simulink model "A320"  (R2023b)
settings: Solver=ode4  StartTime=0.0  StopTime=150  FixedStep=0.001  RelTol=1e-3
values from neighbouring files (symbols this model uses):
  a0 = 340.294    [basedata.m]    (also in basedata.mat; control_design.mat; landing_init.m; landing_plan.mat)
  alpha_CL_table = [ -3.150;  0.000;  0.139;  0.200;  0.260;  0.290;  0.320;  0.500;  3.150 ]    [basedata.m]
  alpha_Cm_table = [ -3.150; -0.800; -0.400; -0.200; -0.100;  0.000;  0.200;  0.230;  0.260;  0.290;  0.310;  0.400;  0.800;  3.150 ]    [basedata.m]
  alpha_Kde_table = [ -3.141593; -0.698132; -0.349066; -0.174533; -0.087266;  0.000000;  0.087266;  0.174533;  0.349066;  0.698132;  3.141593 ]    [basedata.m]
  b_ref = 35.799979    [basedata.m]    (also in basedata.mat = 2; control_design.mat = 2; landing_init.m = 2; landing_plan.mat = 2)
  c_gear = [6.734e4, 1.179e5, 1.179e5]    [basedata.m]    (also in basedata.mat = [8000 14000 14000]; control_design.mat = [8000 14000 14000]; landing_init.m = [0.8e4, 1.4e4, 1.4e4]; landing_plan.mat = [8000 14000 14000])
  c_lat = [9.917e5, 1.852e6, 1.852e6]    [basedata.m]    (also in basedata.mat = [14000 22000 22000]; control_design.mat = [14000 22000 22000]; landing_init.m = [1.4e4, 2.2e4, 2.2e4]; landing_plan.mat = [14000 22000 22000])
  c_ref = S_ref / b_ref    (= 3.41891172618)    [basedata.m]    (also in basedata.mat = 0.9; control_design.mat = 0.9; landing_init.m = 0.9; landing_plan.mat = 0.9)
  c_roll = [0.020, 0.018, 0.018]    [basedata.m]    (also in basedata.mat = [0.02 0.018 0.018]; control_design.mat = [0.02 0.018 0.018]; landing_init.m; landing_plan.mat = [0.02 0.018 0.018])
  CD0 = 0.01865    [basedata.m]    (also in basedata.mat = 0.045; canshujisuan.m = 0.045; control_design.mat = 0.045; landing_init.m = 0.045)
  CL_D0 = CL_D0_clean    (= 0.175)    [basedata.m]
  CL_table = [  0.000;  0.138;  1.320;  1.480;  1.760;  1.750;  1.600;  1.500;  0.000 ]    [basedata.m]
  Clb = 0.554    [basedata.m]    (also in basedata.mat = -0.08; control_design.mat = -0.08; landing_init.m = -0.08; landing_plan.mat = -0.08)
  Clda = -0.291    [basedata.m]    (also in basedata.mat = -0.2; control_design.mat = -0.2; landing_init.m = -0.2; landing_plan.mat = -0.2)
  CLde = -1.652    [basedata.m]    (also in basedata.mat = 0.28; control_design.mat = 0.28; landing_init.m = 0.28; landing_plan.mat = 0.28)
  Cldr = 0.476    [basedata.m]
  Clp = -2.078    [basedata.m]    (also in basedata.mat = -0.7; control_design.mat = -0.7; landing_init.m = -0.7; landing_plan.mat = -0.7)
  CLq = -57.116    [basedata.m]    (also in basedata.mat = 4.5; canshujisuan.m = 3; control_design.mat = 4.5; landing_init.m = 4.5)
  Clr = -2.621    [basedata.m]    (also in basedata.mat = 0.08; control_design.mat = 0.08; landing_init.m = 0.08; landing_plan.mat = 0.08)
  Cm_table = [  0.000; -2.402; -1.861; -0.842; -0.442;  0.000;  1.173;  1.337;  1.489;  1.723;  1.919;  2.276;  2.992;  0.000 ]    [basedata.m]
  Cmde = -11.78    [basedata.m]    (also in basedata.mat = -0.9; control_design.mat = -0.9; landing_init.m = -0.9; landing_plan.mat = -0.9)
  Cmq = -1245.917    [basedata.m]    (also in basedata.mat = -18; control_design.mat = -18; landing_init.m = -18; landing_plan.mat = -18)
  Cnb = 1.296    [basedata.m]    (also in basedata.mat = 0.25; control_design.mat = 0.25; landing_init.m = 0.25; landing_plan.mat = 0.25)
  Cnda = -0.007    [basedata.m]
  Cndr = 1.321    [basedata.m]    (also in basedata.mat = -0.15; control_design.mat = -0.15; landing_init.m = -0.15; landing_plan.mat = -0.15)
  Cnp = 0.742    [basedata.m]    (also in basedata.mat = -0.04; control_design.mat = -0.04; landing_init.m = -0.04; landing_plan.mat = -0.04)
  Cnr = -67.303    [basedata.m]    (also in basedata.mat = -0.45; control_design.mat = -0.45; landing_init.m = -0.45; landing_plan.mat = -0.45)
  CSb = -3.252    [basedata.m]    (also in basedata.mat = -0.7; control_design.mat = -0.7; landing_init.m = -0.7; landing_plan.mat = -0.7)
  CSdr = -2.793    [basedata.m]    (also in basedata.mat = 0.18; control_design.mat = 0.18; landing_init.m = 0.18; landing_plan.mat = 0.18)
  CSr = 17.395    [basedata.m]    (also in basedata.mat = 0.12; control_design.mat = 0.12; landing_init.m = 0.12; landing_plan.mat = 0.12)
  CYp = 1.833    [basedata.m]
  D = 0.5 * rho0 * V^2 * S_ref * CD_current    [canshujisuan.m]
  D0 = 1400    [basedata.m]    (also in basedata.mat; control_design.mat = 800; landing.m; landing_init.m)
  da_max = 0.436332    [basedata.m]    (also in basedata.mat = 25; control_design.mat = 25; landing_init.m = 25; landing_plan.mat = 25)
  da_min = -da_max    (= -0.436332)    [basedata.m]    (also in basedata.mat = -25; control_design.mat = -25; landing_init.m = -25; landing_plan.mat = -25)
  de_max = 0.436332    [basedata.m]    (also in basedata.mat = 25; control_design.mat = 25; landing_init.m = 25; landing_plan.mat = 25)
  de_min = -0.296706    [basedata.m]    (also in basedata.mat = -25; control_design.mat = -25; landing_init.m = -25; landing_plan.mat = -25)
  Delta_CD_flap_tot = 0.1316    [basedata.m]
  Delta_CD_gear = 0.0372    [basedata.m]
  Delta_CD_sp = 0.05775    [basedata.m]
  Delta_CL_flap_tot = 1.867    [basedata.m]
  Delta_CL_sp = -0.466875    [basedata.m]
  Delta_Cm_flap_tot = -0.084    [basedata.m]
  Delta_Cm_gear = 0.0022    [basedata.m]
  Delta_Cm_sp = 0.023    [basedata.m]
  delta_flap_TE_max = 0.698132    [basedata.m]
  delta_flap_TE_tab = [ 0.000000;  0.087266;  0.174533;  0.261799;  0.349066;  0.698132 ]    [basedata.m]
  delta_slat_LE_max = 0.471239    [basedata.m]
  delta_slat_LE_tab = [ 0.000000;  0.314159;  0.314334;  0.383972;  0.384147;  0.471239 ]    [basedata.m]
  DH = pi / 180    (= 0.0174532925199)    [basedata.m]    (also in basedata.mat; control_design.mat; landing_init.m; landing_plan.mat)
  dr_max = 0.436332    [basedata.m]    (also in basedata.mat = 25; control_design.mat = 25; landing_init.m = 25; landing_plan.mat = 25)
  dr_min = -dr_max    (= -0.436332)    [basedata.m]    (also in basedata.mat = -25; control_design.mat = -25; landing_init.m = -25; landing_plan.mat = -25)
  g = 9.80665    [basedata.m]    (also in basedata.mat; canshujisuan.m; control_design.mat; landing_init.m)
  gD_flap_TE_tab = [ 0.000;     0.300;     0.630;     0.850;     0.970;     0.939 ]    [basedata.m]
  gD_slat_LE_tab = [ 1.000;     0.330;     0.630;     0.850;     0.970;     0.939 ]    [basedata.m]
  gL_flap_TE_tab = [ 0.000;     0.010;     1.300;     1.300;     1.170;     1.000 ]    [basedata.m]
  gL_slat_LE_tab = [ 1.000;     1.000;     1.000;     1.000;     1.000;     1.000 ]    [basedata.m]
  ground_z = 0.0    (= 0)    [basedata.m]    (also in basedata.mat; control_design.mat; landing_init.m; landing_plan.mat)
  H_B = 132.622761894    [basedata.mat]    (also in landing_trajectory.m = H_R - R * cos(a1); landingplan.mat)
  H_C = 72.1000994005    [basedata.mat]    (also in landing_trajectory.m = H_R - R * cos(a2); landingplan.mat)
  H_climb_complete = 1000    [control_design.mat]    (also in landing.m; landing_init.m; landing_plan.mat; landingplan.mat)
  H_entry = 1000    [basedata.mat]    (also in landing_trajectory.m; landingplan.mat)
  H_exp = 20    [basedata.mat]    (also in landing_trajectory.m; landingplan.mat)
  HD = 180 / pi    (= 57.2957795131)    [basedata.m]    (also in basedata.mat; control_design.mat; landing_init.m; landing_plan.mat)
  I = [ Ixx, -Ixy, -Ixz ... (first row only)    [basedata.m]    (also in basedata.mat = [120  0  0; 0  480  0; 0  0  520]; control_design.mat = [120  0  0; 0  480  0; 0  0  520]; landing_init.m; landing_plan.mat = [120  0  0; 0  480  0; 0  0  520])
  K_alpha = 7.5375    [basedata.mat]    (also in control_design.m = K_alpha_cruise; control_design.mat; controller.m = 5; landingplan.mat)
  K_GE = 1.0    (= 1)    [basedata.m]
  k_gear = [7.083e6, 2.125e7, 2.125e7]    [basedata.m]    (also in basedata.mat = [100000 300000 300000]; control_design.mat = [100000 300000 300000]; landing_init.m = [1.0e5, 3.0e5, 3.0e5]; landing_plan.mat = [100000 300000 300000])
  k_i_eff = 0.07447685    [basedata.m]
  Kde_table = [ -1.000;     0.050;     0.455;     0.853;     1.007;     1.000;     0.839;     0.693;     0.381;    -0.080;   -1.000 ]    [basedata.m]
  Kn_pitch = -0.120095403309    [basedata.mat]    (also in control_design.m = Kn_pitch_cruise; control_design.mat; controller.m = (2.2*wd^2*g)/(Tr*(wd^2-a24)*V_test*a34); landingplan.mat)
  Kw_pitch = -0.483749055178    [basedata.mat]    (also in control_design.m = Kw_pitch_cruise; control_design.mat; controller.m = -(2*zeta*wd) / a25; landingplan.mat)
  m = 42500.244    [basedata.m]    (also in basedata.mat = 600; canshujisuan.m = 600; control_design.mat = 600; landing_init.m = 600)
  mu_brake = [0.0, 0.55, 0.55]    [basedata.m]    (also in basedata.mat = [0 0.55 0.55]; control_design.mat = [0 0.55 0.55]; landing_init.m; landing_plan.mat = [0 0.55 0.55])
  phi0 = 0    [control_design.mat]    (also in landing.m; landing_init.m; landing_init.mat; landing_plan.mat)
  psi0 = 0    [control_design.mat]    (also in landing.m; landing_init.m; landing_init.mat; landing_plan.mat)
  r_left_b = r_gear_b(:,2)    [basedata.m]    (also in basedata.mat = [-0.333333333333 -0.8 0.65]; control_design.mat = [-0.333333333333 -0.8 0.65]; landing_init.m; landing_plan.mat = [-0.333333333333 -0.8 0.65])
  r_nose_b = r_gear_b(:,1)    [basedata.m]    (also in basedata.mat = [2 0 0.65]; control_design.mat = [2 0 0.65]; landing_init.m; landing_plan.mat = [2 0 0.65])
  r_right_b = r_gear_b(:,3)    [basedata.m]    (also in basedata.mat = [-0.333333333333 0.8 0.65]; control_design.mat = [-0.333333333333 0.8 0.65]; landing_init.m; landing_plan.mat = [-0.333333333333 0.8 0.65])
  rho0 = 1.225    [basedata.m]    (also in basedata.mat; canshujisuan.m; control_design.mat; landing_init.m)
  S_ref = 122.396968    [basedata.m]    (also in basedata.mat = 1.2; canshujisuan.m = 1.2; control_design.mat = 1.2; landing_init.m = 1.2)
  spoiler_max_air = 0.698132    [basedata.m]
  theta0 = 0    [control_design.mat]    (also in landing.m; landing_init.m; landing_init.mat = 0.0523598775598; landing_plan.mat = 0.0523560209424)
  V_app = 128.516392565    [basedata.mat]    (also in landing_trajectory.m = 1.4 * Vs; landingplan.mat)
  V_cruise = 234.072222    [basedata.m]    (also in control_design.m)
  v_eps = 0.20    (= 0.2)    [basedata.m]    (also in basedata.mat; control_design.mat; landing_init.m; landing_plan.mat)
  V_flare = 1.4 * V_stall_full    (= 82.8255554)    [basedata.m]    (also in landing_trajectory.m = V_shallow; takeoff_parameter.m = 1.4 * V_stall_full)
  V_min = 3    [control_design.mat]    (also in landing.m; landing_init.m; landing_plan.mat; landingplan.mat)
  V_shallow = 110.156907913    [basedata.mat]    (also in landing_trajectory.m = 1.2 * Vs; landingplan.mat)
  wheel_radius = [0.381000, 0.584208, 0.584208]    [basedata.m]    (also in basedata.mat = 0.18; control_design.mat = 0.18; landing_init.m = 0.18; landing_plan.mat = 0.18)
  WOW_on = 0.000    (= 0)    [basedata.m]    (also in basedata.mat; control_design.mat; landing_init.m; landing_plan.mat)
  X_landing_start = -11500    [takeoff_parameter.m]
  Xg0 = 0    [control_design.mat]    (also in landing.m = -12000; landing_init.m = -12000; landing_init.mat = -8000; landing_plan.mat = -12000)
  Yg0 = 3    [control_design.mat]    (also in landing.m = 0; landing_init.m = 0; landing_init.mat = 0; landing_plan.mat = 0)
  Zg0 = -10000    [basedata.m]    (also in basedata.mat = -0.8215943; control_design.mat = -0.8215943; landing.m = -1000; landing_init.m = -1000)
undefined symbols (not defined in the file or in its folder): I_xz, I_yz, Ix_Iy, Iy_Iz, Iz_Ix
libraries: simulink x51, matrix_library x19
(part 4 of 4)

== matlab function A320/6DOF-MODEL/动力学/Subsystem3/MATLAB Function ==
  data: phi input; R_bg output; theta input; psi input
function R_bg = ground2body(phi, theta, psi)
T1 = [cos(psi), sin(psi), 0;
     -sin(psi), cos(psi), 0;
      0, 0, 1];
T2 = [cos(theta), 0, -sin(theta);
       0, 1, 0;
      sin(theta), 0, cos(theta)];
T3 = [1, 0, 0;
      0, cos(phi), sin(phi);
      0, -sin(phi), cos(phi)];
R_bg = T3 * T2 * T1;

== matlab function A320/6DOF-MODEL/动力学/dynamics EQ/MATLAB Function ==
  data: alpha input; R_bwind output; beta input
function R_bwind = wind2body(alpha, beta)
T1 = [cos(alpha), 0, sin(alpha);
       0, 1, 0;
       -sin(alpha), 0, cos(alpha)];
T2 = [cos(beta), sin(beta), 0;
       -sin(beta), cos(beta), 0;
       0, 0, 1];
R_wind_b = T2*T1;
R_bwind = R_wind_b';

== matlab function A320/6DOF-MODEL/动力学/dynamics EQ/MATLAB Function1 ==
  data: phi input; R_bg output; theta input; psi input
function R_bg = ground2body(phi, theta, psi)
T1 = [cos(psi), sin(psi), 0;
     -sin(psi), cos(psi), 0;
      0, 0, 1];
T2 = [cos(theta), 0, -sin(theta);
       0, 1, 0;
      sin(theta), 0, cos(theta)];
T3 = [1, 0, 0;
      0, cos(phi), sin(phi);
      0, -sin(phi), cos(phi)];
R_bg = T3 * T2 * T1;

== matlab function A320/6DOF-MODEL/动力学/height/MATLAB Function ==
  data: phi input; R_bg output; theta input; psi input
function R_bg = ground2body(phi, theta, psi)
T1 = [cos(psi), sin(psi), 0;
     -sin(psi), cos(psi), 0;
      0, 0, 1];
T2 = [cos(theta), 0, -sin(theta);
       0, 1, 0;
      sin(theta), 0, cos(theta)];
T3 = [1, 0, 0;
      0, cos(phi), sin(phi);
      0, -sin(phi), cos(phi)];
R_bg = T3 * T2 * T1;

== matlab function A320/6DOF-MODEL/动力学/rotation EQ/MATLAB Function1 ==
  data: w input; wB_X output
function wB_X = wB_X(w) 
p = w(1);
q = w(2);
r = w(3);
wB_X = [0, -r,  q;...
        r,  0, -p;...
       -q,  p,  0];

== matlab function A320/6DOF-MODEL/动力学/起落架模型/MATLAB Function ==
  data: phi input; R_bg output; theta input; psi input
function R_bg = ground2body(phi, theta, psi)
T1 = [cos(psi), sin(psi), 0;
     -sin(psi), cos(psi), 0;
      0, 0, 1];
T2 = [cos(theta), 0, -sin(theta);
       0, 1, 0;
      sin(theta), 0, cos(theta)];
T3 = [1, 0, 0;
      0, cos(phi), sin(phi);
      0, -sin(phi), cos(phi)];
R_bg = T3 * T2 * T1;

== matlab function A320/6DOF-MODEL/动力学/起落架模型/侧向力/Subsystem/MATLAB Function ==
  data: phi input; R_bg output; theta input; psi input
function R_bg = ground2body(phi, theta, psi)
T1 = [cos(psi), sin(psi), 0;
     -sin(psi), cos(psi), 0;
      0, 0, 1];
T2 = [cos(theta), 0, -sin(theta);
       0, 1, 0;
      sin(theta), 0, cos(theta)];
T3 = [1, 0, 0;
      0, cos(phi), sin(phi);
      0, -sin(phi), cos(phi)];
R_bg = T3 * T2 * T1;

== matlab function A320/6DOF-MODEL/动力学/起落架模型/侧向力/Subsystem/主轮侧向方向向量 ==
  data: Cbg input; eg_lat output; eb_lat input
function eg_lat = project_main_lat(Cbg, eb_lat)

e_z = [0; 0; 1];              % 前-右-下坐标系：Z 轴向下
P_g = eye(3) - e_z*e_z.';     % 投影到地面水平面

eg_lat = P_g * Cbg * eb_lat;

n = norm(eg_lat);
if n > 1e-8
    eg_lat = eg_lat / n;
else
    eg_lat = [0; 1; 0];       % 默认地面右向
end

== matlab function A320/6DOF-MODEL/动力学/起落架模型/侧向力/Subsystem/前轮侧向向量 ==
  data: Cbg input; eg_lat output; eb_lat input
function eg_lat = project_lat(Cbg, eb_lat)

e_z = [0; 0; 1];              % 前-右-下坐标系：Z 轴向下
P_g = eye(3) - e_z*e_z.';     % 投影到地面水平面

eg_lat = P_g * Cbg * eb_lat;

n = norm(eg_lat);
if n > 1e-8
    eg_lat = eg_lat / n;
else
    eg_lat = [0; 1; 0];       % 默认地面右向
end

== matlab function A320/6DOF-MODEL/动力学/起落架模型/MATLAB Function1 ==
  data: phi input; R_bg output; theta input; psi input
function R_bg = ground2body(phi, theta, psi)
T1 = [cos(psi), sin(psi), 0;
     -sin(psi), cos(psi), 0;
      0, 0, 1];
T2 = [cos(theta), 0, -sin(theta);
       0, 1, 0;
      sin(theta), 0, cos(theta)];
T3 = [1, 0, 0;
      0, cos(phi), sin(phi);
      0, -sin(phi), cos(phi)];
R_bg = T3 * T2 * T1;

== matlab function A320/6DOF-MODEL/动力学/起落架模型/三轮在地系下的力/摩擦圆限幅/前轮摩擦圆限幅 ==
  data: N input; F_long_out output; F_long input; F_lat input; F_lat_out output
function [F_long_out,F_lat_out]=Dround_saturation_nose(N,F_long,F_lat)
mu=0.65;
F_ALL=sqrt(F_long.^2+F_lat.^2);
if(F_ALL<=mu*N)
    F_long_out=F_long;
    F_lat_out=F_lat;
else
    s=mu*N/F_ALL;
    F_long_out=s*F_long;
    F_lat_out=s*F_lat;
end

== matlab function A320/6DOF-MODEL/动力学/起落架模型/三轮在地系下的力/摩擦圆限幅/主轮摩擦圆限幅左 ==
  data: N input; F_long_out output; F_long input; F_lat input; F_lat_out output
function [F_long_out,F_lat_out]=Dround_saturation_main(N,F_long,F_lat)
mu=0.7;
F_ALL=sqrt(F_long.^2+F_lat.^2);
if(F_ALL<=mu*N)
    F_long_out=F_long;
    F_lat_out=F_lat;
else
    s=mu*N/F_ALL;
    F_long_out=s*F_long;
    F_lat_out=s*F_lat;
end

== matlab function A320/6DOF-MODEL/动力学/起落架模型/三轮在地系下的力/摩擦圆限幅/主轮摩擦圆限幅右 ==
  data: N input; F_long_out output; F_long input; F_lat input; F_lat_out output
function [F_long_out,F_lat_out]=Dround_saturation_main(N,F_long,F_lat)
mu=0.7;
F_ALL=sqrt((F_long).^2+(F_lat).^2);
if(F_ALL<=mu*N)
    F_long_out=F_long;
    F_lat_out=F_lat;
else
    s=mu*N/F_ALL;
    F_long_out=s*F_long;
    F_lat_out=s*F_lat;
end

== matlab function A320/6DOF-MODEL/动力学/起落架模型/法向支反力/MATLAB Function ==
  data: phi input; R_bg output; theta input; psi input
function R_bg = ground2body(phi, theta, psi)
T1 = [cos(psi), sin(psi), 0;
     -sin(psi), cos(psi), 0;
      0, 0, 1];
T2 = [cos(theta), 0, -sin(theta);
       0, 1, 0;
      sin(theta), 0, cos(theta)];
T3 = [1, 0, 0;
      0, cos(phi), sin(phi);
      0, -sin(phi), cos(phi)];
R_bg = T3 * T2 * T1;

== matlab function A320/Guidance/降落阶段/MATLAB Function ==
  settings: updateMethod=DISCRETE  sampleTime=0.001
  data: gamma_cmd output; Flight_Phase input; H_cmd output; X input; h_AGL input; Vg input
 function [gamma_cmd,H_cmd] = landing_longitudinal_guidance(Flight_Phase, X, h_AGL, Vg)
%#codegen

gamma1 = -0.125844364414799;   % 陡下滑角
gamma2 = -0.0261780104712042;  % 浅下滑角

R_round = 8000.0;

L_capture = 600.0;   % 7/8阶段下滑角过渡距离，m
L_shallow = 500.0;   % 10阶段过渡距离，m
L_flare   = 400.0;   % 11阶段拉平过渡距离，m

V_sink_td = 0.3;     % 接地下沉率，m/s

persistent initialized
persistent last_phase
persistent X_prev H_prev gamma_prev
persistent X_enter H_enter gamma_enter
persistent XR HR

if isempty(initialized)
    initialized = true;

    last_phase = Flight_Phase;

    X_prev = X;
    H_prev = h_AGL;
    gamma_prev = 0.0;

    X_enter = X;
    H_enter = h_AGL;
    gamma_enter = 0.0;

    XR = X;
    HR = h_AGL + R_round;
end

dX = X - X_prev;
if dX < 0.0
    dX = 0.0;
end

% 阶段切换时锁存上一阶段的输出，而不是重新用固定边界
if Flight_Phase ~= last_phase
    X_enter = X;
    H_enter = H_prev;
    gamma_enter = gamma_prev;

    if Flight_Phase == 9
        XR = X_enter - R_round * sin(gamma_enter);
        HR = H_enter + R_round * cos(gamma_enter);
    end

    last_phase = Flight_Phase;
    dX = 0.0;
end

if Flight_Phase == 9
    dx = X - XR;
    rad = R_round^2 - dx^2;

    if rad < 1e-6
        rad = 1e-6;
    end

    H_cmd = HR - sqrt(rad);
    gamma_cmd = atan(dx / sqrt(rad));

else
    if Flight_Phase == 6
        gamma_target = 0.0;
        L_use = L_capture;

    elseif Flight_Phase == 7 || Flight_Phase == 8
        gamma_target = gamma1;
        L_use = L_capture;

    elseif Flight_Phase == 10
        gamma_target = gamma2;
        L_use = L_shallow;

    elseif Flight_Phase == 11
        V_use = max(Vg, 1.0);
        s = -V_sink_td / V_use;
        s = min(max(s, -1.0), 1.0);

        gamma_target = asin(s);
        L_use = L_flare;

    else
        gamma_target = 0.0;
        L_use = L_capture;
    end

    alpha = 1.0 - exp(-dX / max(L_use, 1.0));

    gamma_cmd = gamma_prev + alpha * (gamma_target - gamma_prev);
    H_cmd = H_prev + tan(gamma_cmd) * dX;

    if Flight_Phase == 11 && H_cmd < 0.0
        H_cmd = 0.0;
        gamma_cmd = 0.0;
    end
end

X_prev = X;
H_prev = H_cmd;
gamma_prev = gamma_cmd;

== matlab function A320/6DOF-MODEL/动力学/height/MATLAB Function1 ==
  data: phi input; R_bg output; theta input; psi input
function R_bg = ground2body(phi, theta, psi)
T1 = [cos(psi), sin(psi), 0;
     -sin(psi), cos(psi), 0;
      0, 0, 1];
T2 = [cos(theta), 0, -sin(theta);
       0, 1, 0;
      sin(theta), 0, cos(theta)];
T3 = [1, 0, 0;
      0, cos(phi), sin(phi);
      0, -sin(phi), cos(phi)];
R_bg = T3 * T2 * T1;

== stateflow chart A320/Flight Phase Manager/Phase Logic ==
  state Takeoff_Mode
    state Ground_Roll
      en: Flight_Phase = 1;
    state Rotation
      en: Flight_Phase = 2;
    state Liftoff
      en: Flight_Phase = 3;
    state Initial_Climb
      en: Flight_Phase = 4;
    state Climb_Complete
      en: Flight_Phase = 5;
    (default) -> Ground_Roll
    Rotation -> Liftoff : [airborne == true]
    Ground_Roll -> Rotation : [reach_VR==true]
    Liftoff -> Initial_Climb : [safe_climb == true]
    Initial_Climb -> Climb_Complete : [in_cruise==true]
  state Landing_Mode
    state Trajectory_Capture
      en: Flight_Phase = 7;
    state Steep_Glide
      en: Flight_Phase = 8;
    state Round_Flare
      en: Flight_Phase = 9;
    state Approach
      en: Flight_Phase = 6;
    state Roll_out
      en: Flight_Phase = 13;
    state Touchdown
      en: Flight_Phase = 12;
    state Flare
      en: Flight_Phase = 11;
    state Shallow_Glide
      en: Flight_Phase = 10;
    (default) -> Approach
    Approach -> Trajectory_Capture : [Trajectory_capture == true]
    Steep_Glide -> Round_Flare : [in_round==true]
    Trajectory_Capture -> Steep_Glide : [in_steep == true]
    Round_Flare -> Shallow_Glide : [Slight_decline==true]
    Touchdown -> Roll_out : [in_ground==true]
    Flare -> Touchdown : [touch_ground == true]
    Shallow_Glide -> Flare : [in_Flare==true]
  (junction 38) -> Takeoff_Mode [order 1] : [Task_Mode == 1]{Flight_Phase = 0;}
  (default) -> (junction 38)
  (junction 38) -> Landing_Mode [order 2] : {Flight_Phase = 0;}
  Takeoff_Mode -> Landing_Mode : [Task_Mode == 2]
  data: reach_VR input size=1; airborne input size=1; safe_climb input size=1; in_cruise input; Task_Mode input size=1; Trajectory_capture input; in_steep input; in_round input; Slight_decline input; in_Flare input; touch_ground input; in_ground input; Flight_Phase output uint8 size=1 =0

== matlab function A320/controller1/4_Power&V_Ctrl/MATLAB Function2 ==
  data: Vel_g input; dv_err output; axyz input
function dv_err = dv_cal(Vel_g,axyz)
%#codegen

% k_theta = Att_g(1)*pi/180;
% psi = Att_g(2)*pi/180;
% gama = Att_g(3)*pi/180;
% 
% Cg_b = Mx(gama)*Mz(k_theta)*My(psi);
% Cb_g = Cg_b';
vx = Vel_g(1);
vy = Vel_g(2);
vz = Vel_g(3);

ax = axyz(1);
ay = axyz(2);
az = axyz(3);

dv_err = (vx*ax + vy*ay + vz*az)/sqrt(vx^2 + vy^2 + vz^2);
% dv_err = (vx*ax + vz*az)/sqrt(vx^2 + vz^2);
if isnan(dv_err) == 1 
    dv_err = 0;
end

== matlab function A320/6DOF-MODEL/动力学/起落架模型/纵向力/Subsystem/MATLAB Function ==
  data: phi input; R_bg output; theta input; psi input
function R_bg = ground2body(phi, theta, psi)
T1 = [cos(psi), sin(psi), 0;
     -sin(psi), cos(psi), 0;
      0, 0, 1];
T2 = [cos(theta), 0, -sin(theta);
       0, 1, 0;
      sin(theta), 0, cos(theta)];
T3 = [1, 0, 0;
      0, cos(phi), sin(phi);
      0, -sin(phi), cos(phi)];
R_bg = T3 * T2 * T1;

== matlab function A320/6DOF-MODEL/动力学/起落架模型/纵向力/Subsystem/主轮滚动方向向量 ==
  data: Cbg input; eg_long output; eb_long input
function eg_long = project_long(Cbg, eb_long)

e_z = [0; 0; 1];              % 前-右-下坐标系：Z 轴向下
P_g = eye(3) - e_z*e_z.';     % 投影到地面水平面

eg_long = P_g * Cbg * eb_long;

n = norm(eg_long);
if n > 1e-8
    eg_long = eg_long / n;
else
    eg_long = [1; 0; 0];
end

== matlab function A320/6DOF-MODEL/动力学/起落架模型/纵向力/Subsystem/前轮滚动方向向量 ==
  data: Cbg input; eg_long output; eb_long input
function eg_long = project_long(Cbg, eb_long)

e_z = [0; 0; 1];              % 前-右-下坐标系中，Z 轴为下
P_g = eye(3) - e_z*e_z.';     % 投影到地面水平面

eg_long = P_g * Cbg * eb_long;

n = norm(eg_long);
if n > 1e-8
    eg_long = eg_long / n;
else
    eg_long = [1; 0; 0];
end

== matlab function A320/6DOF-MODEL/动力学/起落架模型/起落架三轮质心在地系下位置/MATLAB Function ==
  data: phi input; R_bg output; theta input; psi input
function R_bg = ground2body(phi, theta, psi)
T1 = [cos(psi), sin(psi), 0;
     -sin(psi), cos(psi), 0;
      0, 0, 1];
T2 = [cos(theta), 0, -sin(theta);
       0, 1, 0;
      sin(theta), 0, cos(theta)];
T3 = [1, 0, 0;
      0, cos(phi), sin(phi);
      0, -sin(phi), cos(phi)];
R_bg = T3 * T2 * T1;
